simulink model "PowerTrainModeling"  (R2016a)
settings: Solver=ode3  StartTime=0.0  StopTime=1220  FixedStep=0.1  RelTol=1e-3
libraries: simulink x6
(part 1 of 3)
settings Model: Creator=Admin  LastModifiedBy=karim chamaa
settings DataIOCC: LimitDataPoints=on  SaveFormat=Array  SignalLoggingSaveFormat=ModelDataLogs
settings OptimizationCC: ExpressionDepthLimit=2147483647
settings DebuggingCC: UnderspecifiedInitializationDetection=Classic  MergeDetectMultiDrivingBlocksExec=none  SolverPrmCheckMsg=warning  FcnCallInpInsideContextMsg=UseLocalSettings  StateNameClashWarn=warning
settings HardwareCC: ProdBitPerPointer=32  ProdLargestAtomicFloat=None  ProdIntDivRoundTo=Undefined  ProdEndianess=Unspecified  ProdWordSize=32  ProdHWDeviceType=32-bit Generic
settings ModelReferenceCC: PropagateSignalLabelsOutOfModel=off
settings GRTTargetCC: CombineOutputUpdateFcns=off  GRTInterface=on
settings ConfigComp: CovModelRefEnable=Off  CovSFcnEnable=off

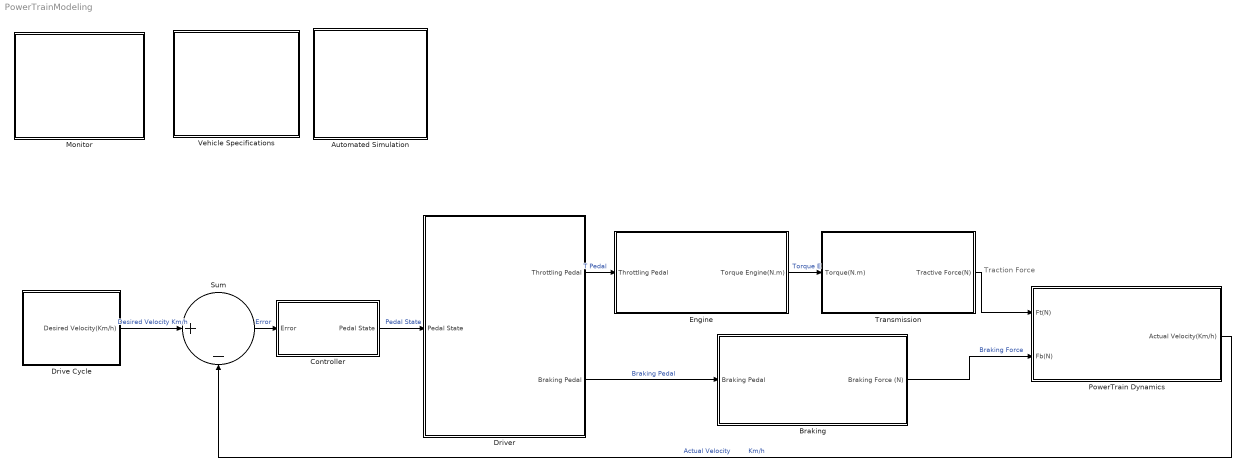
== system PowerTrainModeling ==
  note: Traction Force
  Automated Simulation : Subsystem
      mask Display: image('Clock.png')
  Braking : Subsystem
      mask Display: image('Braking.png')
  Controller : Subsystem
      mask Display: image('Controller.png')
  Drive Cycle : Subsystem
      mask Display: image('DriveCycle.jpg')
  Driver : Subsystem
      mask Display: image('Driver.png')
  "Engine " : Subsystem
      mask Display: image('Engine.jpg')
  Monitor : Subsystem
      mask Display: image('Monitor.jpg')
  "PowerTrain Dynamics " : Subsystem
      mask Display: image('Powertrain.jpg')
  Sum : Sum  Inputs=|+-
  Transmission : Subsystem
      mask Display: image('Transmission.png')
  Vehicle Specifications : Subsystem  mask{M=1392, G=9.81, Alpha=0, Rho=1.2, Af=2, Cd=0.335, Vw=0, Iw=0.4, Rd=0.312, i0=3, Ie=0.1, Option=1, GbE=0.95, DE=0.97, PL=300, FD=0.74, ROG1=3.62, ROG2=2.22, ROG3=1.51, ROG4=1.08, ROG5=0.85, EIS=750, EMS=6000}
      mask prompts: M "Total Mass(Kg)"; G "Gravitational Acceleration(m/s^2)"; Alpha "Gradient(degree)"; Rho "Air Density (Kg/m^3)"; Af "Frontal Surface Area(m^2)"; Cd "Drag Coefficiant"; Vw "Wind Speed (m/s)"; Iw "Four Wheels Inertia(Kg.m^2)"; Rd "Wheel Radius(m)"; i0 "Final Drive Ratio"; Ie "Engine Inertia(Kg.m^2)"; Option "1-Nedc(1220),2-EUDC(400),3-UDC(247)"; GbE "GearBox Efficiency"; DE "Differential Efficiency"; PL "Power Loss(W)"; FD "Fuel Density(Kg/L)"; ROG1 "Ratio Of Gear 1"; ROG2 "Ratio Of Gear 2"; ROG3 "Ratio Of Gear 3"; ROG4 "Ratio Of Gear 4"; ROG5 "Ratio Of Gear 5"; EIS "Engine Idle Speed(RPM)"; EMS "Engine Maximum Speed(RPM)"
      mask Display: image('Specs.jpg')
  wires:
  "Engine "/1(Torque Engine(N.m)) -> Transmission/1(Torque(N.m))  "Torque E"
  Driver/1(Throttling Pedal) -> "Engine "/1(Throttling Pedal)  "T Pedal"
  Driver/2(Braking Pedal) -> Braking/1(Braking Pedal)  "Braking Pedal"
  Controller/1(Pedal State) -> Driver/1("Pedal State ")  "Pedal State"
  Sum/1 -> Controller/1(Error)  "Error"
  Transmission/1(Tractive Force(N)) -> "PowerTrain Dynamics "/1(Ft(N))
  Braking/1(Braking Force (N)) -> "PowerTrain Dynamics "/2(Fb(N))  "Braking Force"
  "PowerTrain Dynamics "/1(" Actual Velocity(Km/h)") -> Sum/2  "Actual Velocity         Km/h"
  Drive Cycle/1(Desired Velocity(Km/h)) -> Sum/1  "Desired Velocity Km/h"

== system PowerTrainModeling/Automated Simulation ==
  Clock : Clock
  EUDC cycle : Constant  Value=400
  NEDC cylce : Constant  Value=1220
  Relational Operator : RelationalOperator  OutDataTypeStr=boolean
  Stop Simulation : Stop
  "Switch Depend On Option Selected " : MultiPortSwitch
  UDC cyle : Constant  Value=247
  wires:
  [Option] -> "Switch Depend On Option Selected "/1
  NEDC cylce/1 -> "Switch Depend On Option Selected "/2
  Clock/1 -> Relational Operator/1
  "Switch Depend On Option Selected "/1 -> Relational Operator/2
  EUDC cycle/1 -> "Switch Depend On Option Selected "/3
  UDC cyle/1 -> "Switch Depend On Option Selected "/4
  Relational Operator/1 -> Stop Simulation/1

== system PowerTrainModeling/Braking ==
  Braking Pedal : Inport
  Maximum Braking Force(N) : Constant  Value=5000
  Product : Product
  Scope : Scope
  Braking Force (N) : Outport
  wires:
  Braking Pedal/1 -> Product/1
  Product/1 -> Scope/1, Braking Force (N)/1  "Braking Force (N)"
  Maximum Braking Force(N)/1 -> Product/2

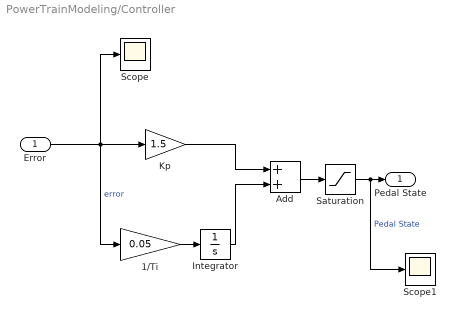
== system PowerTrainModeling/Controller ==
  Error : Inport
  1/Ti : Gain  Gain=0.05
  Add : Sum
  Integrator : Integrator
  Kp : Gain  Gain=1.5
  Saturation : Saturate  UpperLimit=1  LowerLimit=-1
  Scope : Scope
  Scope1 : Scope
  Pedal State : Outport
  wires:
  Add/1 -> Saturation/1
  Integrator/1 -> Add/2
  1/Ti/1 -> Integrator/1
  Kp/1 -> Add/1
  Error/1 -> Scope/1, 1/Ti/1, Kp/1  "error"
  Saturation/1 -> Scope1/1, Pedal State/1  "Pedal State"
